simulink model "MBD_APPLI_JOC2017"  (R2016a)
settings: Solver=FixedStepDiscrete  StartTime=0.0  StopTime=inf  FixedStep=0.001  RelTol=1e-3
InitFcn:
  | Param
values from neighbouring files (symbols this model uses):
  H_MOV_LEV = 1.0    (= 1)    [Param.m]
  H_TAG_DIS = 2.35    [Param.m]
  HMAN_INI_X = -154    [Param.m]
  HMAN_INI_Z = 397.5    [Param.m]
  HMAN_VEL_K = 5.00107    [Param.m]
  MYCAR_INI_X = -194    [Param.m]
  MYCAR_INI_Z = 390    [Param.m]
  SIKI_1 = 10.0    (= 10)    [Param.m]
  SIKI_2 = 7.0    (= 7)    [Param.m]
  SIKI_3 = 4.0    (= 4)    [Param.m]
  SIKI_4 = 5.0    (= 5)    [Param.m]
  SIKI_5 = 2.0    (= 2)    [Param.m]
libraries: dspnetwork x6, realtime_pacer_lib x1
settings Model: ModifiedByFormat=mbd_app  Creator=mbd_app  LastModifiedBy=mbd_app
settings DebuggingCC: AlgebraicLoopMsg=none

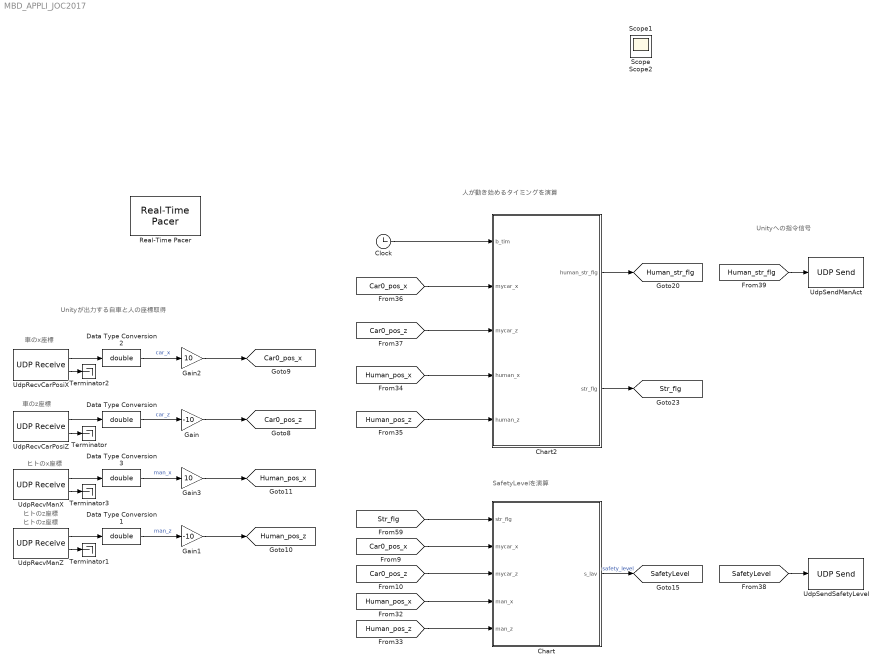
== system MBD_APPLI_JOC2017 ==
  note: 車のz座標
  note: ヒトのz座標
  note: 車のx座標
  note: ヒトのx座標
  note: Unityが出力する自車と人の座標取得
  note: ヒトのz座標
  note: 人が動き始めるタイミングを演算
  note: Unityへの指令信号
  note: SafetyLevelを演算
  Chart : Stateflow chart  TreatAsAtomicUnit=on
  Chart2 : Stateflow chart  TreatAsAtomicUnit=on
  Clock : Clock
  Data Type Conversion{,1..3} (4 alike) : DataTypeConversion  OutDataTypeStr=double
  Gain : Gain  Gain=-10
  Gain1 : Gain  Gain=-10
  Gain2 : Gain  Gain=10
  Gain3 : Gain  Gain=10
  Real-Time Pacer : realtime_pacer_lib/Real-Time Pacer  simTimePerRealTime=1
  Terminator{,1..3} (4 alike) : Terminator
  UdpRecvCarPosiX : dspnetwork/UDP Receive  localURL='0.0.0.0'  localPort=3333  remoteURL='localhost'  remotePort=-1  recvBufferSize=4  dims=1  signalDatatype=single  isVarSize=off  showBlockingTime=off  blockingTime=0  sampletime=-1  blockPlatform=[]
  UdpRecvCarPosiZ : dspnetwork/UDP Receive  localURL='0.0.0.0'  localPort=3334  remoteURL='localhost'  remotePort=-1  recvBufferSize=4  dims=1  signalDatatype=single  isVarSize=off  showBlockingTime=off  blockingTime=0  sampletime=-1  blockPlatform=[]
  UdpRecvManX : dspnetwork/UDP Receive  localURL='0.0.0.0'  localPort=3335  remoteURL='localhost'  remotePort=-1  recvBufferSize=4  dims=1  signalDatatype=single  isVarSize=off  showBlockingTime=off  blockingTime=0  sampletime=-1  blockPlatform=[]
  UdpRecvManZ : dspnetwork/UDP Receive  localURL='0.0.0.0'  localPort=3336  remoteURL='localhost'  remotePort=-1  recvBufferSize=4  dims=1  signalDatatype=single  isVarSize=off  showBlockingTime=off  blockingTime=0  sampletime=-1  blockPlatform=[]
  UdpSendManAct : dspnetwork/UDP Send  remoteURL='localhost'  remotePort=43395  localURL='0.0.0.0'  localPortSource=Automatically determine  localPort=-1  sampletime=-1  blockPlatform=[]  separateLengthPort=0
  UdpSendSafetyLevel : dspnetwork/UDP Send  remoteURL='localhost'  remotePort=43385  localURL='0.0.0.0'  localPortSource=Automatically determine  localPort=-1  sampletime=-1  blockPlatform=[]  separateLengthPort=0
  Scope : Scope
  Scope1 : Scope
  Scope2 : Scope
  tag scope: Car0_pos_x=global, Car0_pos_z=global, Human_pos_x=global, Human_pos_z=global, Human_str_flg=global, SafetyLevel=global, Str_flg=global
  wires:
  UdpRecvCarPosiX/1 -> Data Type Conversion2/1
  UdpRecvCarPosiZ/1 -> Data Type Conversion/1
  UdpRecvManX/1 -> Data Type Conversion3/1
  UdpRecvManZ/1 -> Data Type Conversion1/1
  Gain/1 -> [Car0_pos_z]
  Gain1/1 -> [Human_pos_z]
  UdpRecvCarPosiZ/2 -> Terminator/1
  UdpRecvManZ/2 -> Terminator1/1
  UdpRecvCarPosiX/2 -> Terminator2/1
  UdpRecvManX/2 -> Terminator3/1
  Chart/1(s_lav) -> [SafetyLevel]  "safety_level"
  [Car0_pos_x] -> Chart/2(mycar_x)
  [Car0_pos_z] -> Chart/3(mycar_z)
  [Human_pos_x] -> Chart/4(man_x)
  Clock/1 -> Chart2/1(b_tim)
  [Human_str_flg] -> UdpSendManAct/1
  [SafetyLevel] -> UdpSendSafetyLevel/1
  [Car0_pos_x] -> Chart2/2(mycar_x)
  [Human_pos_x] -> Chart2/4(human_x)
  [Car0_pos_z] -> Chart2/3(mycar_z)
  [Human_pos_z] -> Chart2/5(human_z)
  Gain3/1 -> [Human_pos_x]
  Gain2/1 -> [Car0_pos_x]
  Data Type Conversion2/1 -> Gain2/1  "car_x"
  Data Type Conversion/1 -> Gain/1  "car_z"
  Data Type Conversion3/1 -> Gain3/1  "man_x"
  Data Type Conversion1/1 -> Gain1/1  "man_z"
  Chart2/1(human_str_flg) -> [Human_str_flg]
  Chart2/2(str_flg) -> [Str_flg]
  [Str_flg] -> Chart/1(str_flg)
  [Human_pos_z] -> Chart/5(man_z)

== stateflow chart MBD_APPLI_JOC2017/Chart2 ==
  (default) -> (junction 203)
  (junction 203) -> (junction 205) [order 2]
  (junction 203) -> (junction 204) [order 1] : % Unityの実行時間[sec]をげっと初回
      | % MATLABとUnityの連成開始
      | [(str_flg == false) &  ((abs(mycar_x - MYCAR_INI_X)) < 0.1) & (abs(human_x - HMAN_INI_X) < 0.1)]
      |  {
      |   str_flg = 1.0;
      | }
  (junction 205) -> (junction 222)
  (junction 222) -> (junction 250) [order 2]
  (junction 204) -> (junction 222)
  (junction 250) -> (junction 252) : % Unityからの入力情報が更新されない対応
      | {
      |  mycar_x_o = mycar_x;
      |  mycar_z_o = mycar_z;
      |  mycar_tch_tim = mycar_tch_tim_o;
      | }
  (junction 222) -> (junction 225) [order 1] : % 自車と人の情報更新タイミングが一致していないので、分ける。
      | % ここでは、自車の情報をUnityから取得して位置や速度を演算する。
      | % Unityからの入力情報が更新されたら演算
      | [(str_flg_o == true) & (mycar_x ~= mycar_x_o)]
      |  {
      |   % 演算時間更新
      |   b_tim_o = b_tim;
      |   % 自車の瞬時移動距離[m]
      |   mycar_mov = sqrt(((mycar_z - mycar_z_o)^2) + ((mycar_x - mycar_x_o)^2));
      |   % 自車の車速[m/sec]
      |   mycar_vel = mycar_mov / 0.01;
      |   % Unityからの入力情報が更新されない際の情報すとっく
      |   mycar_x_o = mycar_x;
      |   mycar_z_o = mycar_z;
      |   mycar_mov_o = mycar_mov;
      |   mycar_vel_o = mycar_vel;
      |  }
  (junction 225) -> (junction 236) [order 2]
  (junction 225) -> (junction 234) [order 1] : % 自車が人をX方向に通過 or 人が自車をz方向に通過_後
      | [(human_x < mycar_x) || (human_z < mycar_z)]
      |  {
      |   % 自車が人と接触するポイントまでの時間[sec]
      |   mycar_tch_tim = 0.0;
      |   mycar_tch_tim_o = 0.0;
      |  }
  (junction 236) -> (junction 238) : % 自車が人をX方向に通過 or 人が自車をz方向に通過_前
      |   % 自車が人と接触するポイントまでの距離[m]
      |  {
      |   mycar_tch_dis = human_x - mycar_x;
      |  }
  (junction 238) -> (junction 242) [order 2]
  (junction 238) -> (junction 240) [order 1] : % 自車が人と接触するポイントまでの時間[sec]
      | % 初期値=50.0secでmaxガード
      | [50.0 <= (mycar_tch_dis / mycar_vel)]
      |  {
      |   mycar_tch_tim = 50.0;
      |   mycar_tch_tim_o = mycar_tch_tim;
      |  }
  (junction 242) -> (junction 244) : % 通常演算
      |  {
      |   mycar_tch_tim = mycar_tch_dis / mycar_vel;
      |   mycar_tch_tim_o = mycar_tch_tim;
      |  }
  (junction 234) -> (junction 240)
  (junction 240) -> (junction 244)
  (junction 244) -> (junction 252)
  (junction 252) -> (junction 266) : % 自車が人をX方向に通過 or 人が自車をz方向に通過_前
      |  {
      |   % 人が自車と接触するポイントまでの距離[m]
      |   human_tch_dis = human_z - mycar_z + H_TAG_DIS;
      |   % 人が自車と接触するポイントまでの時間[sec]
      |   human_tch_tim = human_tch_dis / (HMAN_VEL_K * H_MOV_LEV);
      |  }
  (junction 266) -> (junction 273) [order 2]
  (junction 266) -> (junction 271) [order 1] : % 人の飛出し開始フラグ
      | [mycar_tch_tim <= human_tch_tim]
      |  { human_str_flg = H_MOV_LEV; }
  (junction 273) -> (junction 277) : { human_str_flg = human_str_flg_o; }
  (junction 271) -> (junction 277)
  (junction 277) -> (junction 283) : % 更新
      | {
      |   str_flg_o = str_flg;
      |   human_str_flg_o = human_str_flg;
      | }
  data: human_str_flg output =0; str_flg output =0; b_tim input; mycar_x input; mycar_z input; human_x input; human_z input; b_tim_o local =0; human_str_flg_o local =0; human_x_o local =HMAN_INI_X; human_x_o1 local =0; human_z_o local =HMAN_INI_Z; mov_o1 local =0; mov_o2 local =0; mov_o3 local =0; mov_o4 local =0; mov_o5 local =0; mov_ox local =0; mycar_mov_o local =0; mycar_tmov_o1 local =50; mycar_vel_o local =0; h_vel_o1 local =0; h_vel_o2 local =0; h_vel_o3 local =0; h_vel_o4 local =0; h_vel_o5 local =0; mycar_x_o local =MYCAR_INI_X; mycar_z_o local =MYCAR_INI_Z; H_MOV_LEV parameter; H_TAG_DIS parameter; str_tim local =0; mycar_tch_dis_o local =50; mycar_tch_tim_o local =10; human_tch_dis_o local =10; HMAN_VEL_K parameter; human_tch_tim_o local =10; human_vel_o local =1.5; mycar_tmov local double =0; MYCAR_INI_X parameter; MYCAR_INI_Z parameter; HMAN_INI_X parameter; HMAN_INI_Z parameter; str_flg_o local =0; hb_tim local =0; ope_tim local; mycar_mov local =0; mycar_vel local =0; mycar_tch_dis local =100; mycar_tch_tim local [..50] =50; human_tch_dis local; human_tch_tim local =30; human_vel local =0

== stateflow chart MBD_APPLI_JOC2017/Chart ==
  (default) -> (junction 5)
  (junction 5) -> (junction 7) [order 2]
  (junction 5) -> (junction 16) [order 1] : [(str_flg == true) &...
      |  ((man_x - mycar_x) <= SIKI_1)  &...
      |  ((man_z - mycar_z) <= SIKI_4) &...
      |   ((mycar_z - man_z) <= SIKI_5)
      | ]
  (junction 7) -> (junction 58) : {s_lav = 0.0;}
  (junction 16) -> (junction 56) [order 2]
  (junction 16) -> (junction 15) [order 1] : [(man_x - mycar_x) <= SIKI_3]
      | {s_lav = 3.0;}
  (junction 56) -> (junction 24)
  (junction 24) -> (junction 30) [order 2]
  (junction 24) -> (junction 26) [order 1] : [(man_x - mycar_x) <= SIKI_2]
      | {s_lav = 2.0;}
  (junction 30) -> (junction 32) : {s_lav = 1.0;}
  (junction 15) -> (junction 26)
  (junction 26) -> (junction 32)
  (junction 32) -> (junction 58)
  data: str_flg input; mycar_x input; mycar_z input; man_x input; man_z input; s_lav output; SIKI_3 parameter double; SIKI_2 parameter; SIKI_1 parameter; SIKI_4 parameter; SIKI_5 parameter
